simulink model "ExerciseModel_18072025"  (R2025a)
settings: Solver=ode4  StartTime=0.0  StopTime=tsim  FixedStep=1  RelTol=1e-3
model workspace (MAT data in the model file):
  step_size = 1
values from neighbouring files (symbols this model uses):
  A_w = [cosd(beta1)*sind(alfa1)  -cosd(beta2)*sind(alfa2) -cosd(beta3)*sind(alfa3) cosd(beta4)*sind(alfa4) ... (first row only)    [initfun_18072025.m]    (also in initfun_18072025_nogyro.m)
  A_wP = pinv(A_w)    [initfun_18072025.m]    (also in initfun_18072025_nogyro.m)
  ARW = deg2rad(0.23)/sqrt(3600)    [initfun_18072025.m]
  Bias = deg2rad(1)/3600    [initfun_18072025.m]
  C_d = 2.2    [initfun_18072025.m]    (also in initfun_18072025_nogyro.m)
  d_max = 0.29    [initfun_18072025.m]    (also in initfun_18072025_nogyro.m)
  d_min = 0    [initfun_18072025.m]    (also in initfun_18072025_nogyro.m)
  ET0 = cspice_str2et(Date_UTC)    [initfun_18072025.m]    (also in initfun_18072025_nogyro.m)
  FOV = 166    [initfun_18072025.m]    (also in initfun_18072025_nogyro.m)
  G_earth = 6.6742e-11    [initfun_18072025.m]    (also in initfun_18072025_nogyro.m)
  init_state = [initial_position,initial_velocity,ang_vel_init2,quat_0]'    [initfun_18072025.m]    (also in initfun_18072025_nogyro.m)
  K = [F Z(:); Z(:)' sigma]    [Gain_matrix.m]    (also in QUEST.m = Gain_matrix(V',W',a); initfun_18072025.m = schmidt(nmax, mmax); initfun_18072025_nogyro.m = schmidt(nmax, mmax))
  K_dp = K_d_pitch_1    [evaluate_gains.m]    (also in evaluate_gains_nogyro.m)
  K_dr = K_d_roll_1    [evaluate_gains.m]    (also in evaluate_gains_nogyro.m)
  K_dy = K_d_yaw_1    [evaluate_gains.m]    (also in evaluate_gains_nogyro.m)
  K_pp = K_p_pitch_1    [evaluate_gains.m]    (also in evaluate_gains_nogyro.m; initfun_18072025_nogyro.m = K_pp/2)
  K_pr = K_p_roll_1    [evaluate_gains.m]    (also in evaluate_gains_nogyro.m; initfun_18072025.m = K_pr*1.8)
  K_py = K_p_yaw_1    [evaluate_gains.m]    (also in evaluate_gains_nogyro.m; initfun_18072025.m = K_py*10)
  m_earth = 5.9736e24    (= 5.9736e+24)    [initfun_18072025.m]    (also in initfun_18072025_nogyro.m)
  Magnetic_dipole = [0.1; 0.1;  0.1]    [initfun_18072025.m]    (also in initfun_18072025_nogyro.m)
  Magnetometers_number = 2    [initfun_18072025.m]    (also in initfun_18072025_nogyro.m)
  Mean_cart_Mag = 0    [initfun_18072025.m]    (also in initfun_18072025_nogyro.m)
  MeanangularSun = 0    [initfun_18072025.m]    (also in initfun_18072025_nogyro.m)
  mmax = 3    [initfun_18072025.m]    (also in initfun_18072025_nogyro.m)
  nmax = 3    [initfun_18072025.m]    (also in initfun_18072025_nogyro.m)
  omegaOrb = [0;-2*pi/P;0]    [initfun_18072025.m]    (also in initfun_18072025_nogyro.m)
  P_prev = [P_dg, zeros(3,3) ... (first row only)    [initfun_18072025.m]    (also in initfun_18072025_nogyro.m)
  P_sun = 4.56e-6    (= 4.56e-06)    [initfun_18072025.m]    (also in initfun_18072025_nogyro.m)
  Q = [eye(3,3).*Qattitudefactor zeros(3,3) ... (first row only)    [initfun_18072025.m]    (also in initfun_18072025_nogyro.m)
  R_B = (Sigma_cart_Mag)^2    (= 2.77777777778e-16)    [initfun_18072025.m]    (also in initfun_18072025_nogyro.m)
  r_earth = 6371e3    (= 6371000)    [initfun_18072025.m]    (also in initfun_18072025_nogyro.m)
  R_G = ARW^2    [initfun_18072025.m]
  R_SS = (SigmaangularSun*pi/180)^2    (= 3.04617419787e-06)    [initfun_18072025.m]    (also in initfun_18072025_nogyro.m)
  RWs_Inertia = diag([9.0718e-06, 9.0718e-06, 9.0718e-06, 9.0718e-06])    [initfun_18072025.m]    (also in initfun_18072025_nogyro.m)
  RWs_Inertia_Inv = inv(RWs_Inertia)    [initfun_18072025.m]    (also in initfun_18072025_nogyro.m)
  Sat_Inertia = diag([6.295, 1.644, 5.462]*10^-1)    [initfun_18072025.m]    (also in initfun_18072025_nogyro.m)
  Sat_mass = 12.172    [initfun_18072025.m]    (also in initfun_18072025_nogyro.m)
  Sigma_cart_Mag = (50*10^-9)/3    (= 1.66666666667e-08)    [initfun_18072025.m]    (also in initfun_18072025_nogyro.m)
  SigmaangularSun = 0.1    [initfun_18072025.m]    (also in initfun_18072025_nogyro.m)
  Sun_sensors = zeros(3, SS_number)    [initfun_18072025.m]    (also in initfun_18072025_nogyro.m)
  threshold_omega = omega_max * 0.8    (= 837.7580408)    [initfun_18072025.m]    (also in initfun_18072025_nogyro.m)
  x_prev = x0    [initfun_18072025.m]    (also in initfun_18072025_nogyro.m)
undefined symbols (not defined in the file or in its folder): DiscIntNeverNeededParam, G, H, IAU, juliandate, quat_feed_reg, Sat_Aeromodel_det
libraries: matrix_library x9, vrlib x2, aerolibtransform2 x1
(part 2 of 3)

== system ExerciseModel_18072025/External Disturbance Torques/Magnetic Torque ==
  POS_ECI [km] : Inport
  R(IRF->BRF) : Inport  Port=2
  Cross Product : matrix_library/Cross Product
  Earth magnetc Field : Subsystem
  m : Constant  Value=Magnetic_dipole
  T_mag : Outport
  B : Outport  Port=2
  IRF Earth magnetic field (T) : Outport  Port=3
  wires:
  POS_ECI [km]/1 -> Earth magnetc Field/1(R_ECI)
  Earth magnetc Field/1("BRF Earth magnetic field (T)  ") -> Cross Product/2, B/1
  m/1 -> Cross Product/1
  Cross Product/1 -> T_mag/1
  R(IRF->BRF)/1 -> Earth magnetc Field/2(R(IRF->BRF))
  Earth magnetc Field/2(IRF Earth magnetic field (T)) -> IRF Earth magnetic field (T)/1

== system ExerciseModel_18072025/External Disturbance Torques/SRP_torque_evaluation ==
  Sdir_eci_vec : Inport
  R_ECIBRF : Inport  Port=2
  eclipse_flag : Inport  Port=3
  Constant : Constant  Value=P_sun
  SRP1 : MATLAB Function  TreatAsAtomicUnit=on  SystemSampleTime=step_size
  To Workspace : ToWorkspace  VariableName=srp_torque  SaveFormat=Timeseries  SampleTime=-1
  To Workspace1 : ToWorkspace  VariableName=torque_contrib  SaveFormat=Timeseries  SampleTime=-1
  torque_SRP : Outport
  wires:
  Sdir_eci_vec/1 -> SRP1/1(Sdir_ECI_vec)
  R_ECIBRF/1 -> SRP1/2(R_ECIBRF)
  SRP1/1(torque) -> To Workspace/1, torque_SRP/1
  eclipse_flag/1 -> SRP1/3(eclipse_flag)
  Constant/1 -> SRP1/4(P_sun)
  SRP1/2(torque_contribution) -> To Workspace1/1

== system ExerciseModel_18072025/Performance Block /Altitude Check ==
  In1 : Inport
  Constant : Constant  Value=r_earth*10^-3
  Dot Product : DotProduct  OutDataTypeStr=Inherit: Inherit via internal rule
  Scope : Scope
      settings: ActiveDisplayYMinimum=615.9620311742791  ActiveDisplayYMaximum=646.34171943145168
  Square Root : Sqrt
  Subtract : Sum  Inputs=+-
  wires:
  In1/1 -> Dot Product/1, Dot Product/2
  Constant/1 -> Subtract/2
  Square Root/1 -> Subtract/1
  Dot Product/1 -> Square Root/1
  Subtract/1 -> Scope/1

== system ExerciseModel_18072025/Performance Block /Mo ==
  X (km) [ECI] : Inport
  V (km/s) [ECI] : Inport  Port=2
  MATLAB Function : MATLAB Function  TreatAsAtomicUnit=on
  Transpose : Math  Operator=transpose
  Out1 : Outport
  wires:
  Transpose/1 -> Out1/1
  MATLAB Function/1(Mo) -> Transpose/1
  X (km) [ECI]/1 -> MATLAB Function/1(X)
  V (km/s) [ECI]/1 -> MATLAB Function/2(V)

== system ExerciseModel_18072025/Actuators/RW simplified model/Subsystem ==
  omega_old : Inport
  Constant1 : Constant  Value=RWs_Inertia
  Constant2 : Constant  Value=A_w
  Demux2 : Demux
  Matrix Multiply1 : Product  Multiplication=Matrix(*)
  Matrix Multiply2 : Product  Multiplication=Matrix(*)
  Scope1 : Scope  NumInputPorts=4
      settings: ActiveDisplayYMinimum=-0.0627  ActiveDisplayYMaximum=0.0755
  To Workspace : ToWorkspace  VariableName=h_wheels2  SaveFormat=Structure  SampleTime=-1
      settings: Save2DSignal=2-D array (concatenate along first dimension)
  To Workspace2 : ToWorkspace  VariableName=h_wheels3  SaveFormat=Structure  SampleTime=-1
      settings: Save2DSignal=2-D array (concatenate along first dimension)
  Transpose : Math  Operator=transpose
  hw_w : Outport
  Hw_4w : Outport  Port=2
  wires:
  Transpose/1 -> To Workspace/1
  Matrix Multiply2/1 -> hw_w/1
  Constant2/1 -> Matrix Multiply2/1
  Demux2/1 -> Scope1/1
  Demux2/4 -> Scope1/4
  Constant1/1 -> Matrix Multiply1/1
  Matrix Multiply1/1 -> Matrix Multiply2/2, To Workspace2/1, Transpose/1, Hw_4w/1, Demux2/1
  Demux2/2 -> Scope1/2
  Demux2/3 -> Scope1/3
  omega_old/1 -> Matrix Multiply1/2

== system ExerciseModel_18072025/Discrete Drag in ECI/DRAG FORCE IN ORF [N]/AREA LOOK-UP ==
  roll : Inport
  pitch angle : Inport  Port=2
  yaw angle : Inport  Port=3
  MATLAB Function : MATLAB Function  TreatAsAtomicUnit=on
  Merge : Merge
  Scope2 : Scope
      settings: ActiveDisplayYMinimum=-0.588573963748372  ActiveDisplayYMaximum=0.52172797483263089  DataLoggingVariableName=ScopeData26
  Subsystem : Subsystem
  Subsystem1 : Subsystem
  Area : Outport
  wires:
  Merge/1 -> Area/1, Scope2/1
  Subsystem1/1(Area) -> Merge/2
  MATLAB Function/2(out2) -> Subsystem1/Enable
  MATLAB Function/1(out1) -> Subsystem/Enable
  yaw angle/1 -> Subsystem/3(yaw angle), Subsystem1/3(yaw angle), MATLAB Function/3(yaw_angle)
  pitch angle/1 -> MATLAB Function/2(pitch_angle), Subsystem/2(pitch angle), Subsystem1/2(pitch angle)
  roll/1 -> MATLAB Function/1(roll_angle), Subsystem/1(roll), Subsystem1/1(roll)
  Subsystem/1(Area) -> Merge/1

== system ExerciseModel_18072025/External Disturbance Torques/AeroTorque in BRF/TORQUE FACTOR ==
  roll : Inport
  pitch angle : Inport  Port=2
  yaw angle : Inport  Port=3
  MATLAB Function : MATLAB Function  TreatAsAtomicUnit=on
  Merge : Merge
  Subsystem : Subsystem
  Subsystem1 : Subsystem
  T_comp : Outport
  wires:
  Subsystem1/1(T_components) -> Merge/2
  Merge/1 -> T_comp/1
  Subsystem/1(T_components) -> Merge/1
  MATLAB Function/2(out2) -> Subsystem1/Enable
  MATLAB Function/1(out1) -> Subsystem/Enable
  yaw angle/1 -> MATLAB Function/3(yaw_angle), Subsystem/3(yaw angle), Subsystem1/3(yaw angle)
  pitch angle/1 -> MATLAB Function/2(pitch_angle), Subsystem/2(pitch angle), Subsystem1/2(pitch angle)
  roll/1 -> MATLAB Function/1(roll_angle), Subsystem/1(roll), Subsystem1/1(roll)

== system ExerciseModel_18072025/External Disturbance Torques/Magnetic Torque/Earth magnetc Field ==
  R_ECI : Inport
  R(IRF->BRF) : Inport  Port=2
  Clock : Clock
  Direction Cosine Matrix ECI to ECEF : aerolibtransform2/Direction Cosine Matrix ECI to ECEF  red=IAU-2000/2006  year=2025  month=July  day=23  hour=8  min=30  sec=0  deltaT=Sec  errorflag=Error  extraparamflag=off
      settings: AttributesFormatString=%<red>
  "Earth magnetic field " : MATLAB Function  TreatAsAtomicUnit=on
  G : Constant  Value=G  VectorParams1D=off
  H : Constant  Value=H  VectorParams1D=off
  K : Constant  Value=K  VectorParams1D=off
  Math Function : Math  Operator=transpose  SignedPower=on
  Matrix Multiply : Product  Multiplication=Matrix(*)
  Matrix Multiply1 : Product  Multiplication=Matrix(*)
  Matrix Multiply2 : Product  Multiplication=Matrix(*)
  "Maximum degree of harmonics " : Constant  Value=mmax
  "Maximum order of harmonics " : Constant  Value=nmax
  Reshape : Reshape  OutputDimensionality=Column vector (2-D)
  Reshape1 : Reshape  OutputDimensionality=Column vector (2-D)
  Scope : Scope
      settings: ActiveDisplayYMinimum=-5.8566873314651838E-5  ActiveDisplayYMaximum=5.7983261253001576E-5  DataLoggingVariableName=ScopeData41
  "BRF Earth magnetic field (T)  " : Outport
  IRF Earth magnetic field (T) : Outport  Port=2
  wires:
  R(IRF->BRF)/1 -> Matrix Multiply/1
  Matrix Multiply/1 -> "BRF Earth magnetic field (T)  "/1, Scope/1
  Math Function/1 -> Matrix Multiply1/1
  "Earth magnetic field "/1(B) -> Reshape1/1
  Matrix Multiply2/1 -> "Earth magnetic field "/1(r_ECEF)
  Direction Cosine Matrix ECI to ECEF/1 -> Matrix Multiply2/1, Math Function/1
  Matrix Multiply1/1 -> Matrix Multiply/2, IRF Earth magnetic field (T)/1
  Clock/1 -> Direction Cosine Matrix ECI to ECEF/1
  H/1 -> "Earth magnetic field "/6(H)
  "Maximum order of harmonics "/1 -> "Earth magnetic field "/2(nmax)
  "Maximum degree of harmonics "/1 -> "Earth magnetic field "/3(mmax)
  G/1 -> "Earth magnetic field "/5(G)
  K/1 -> "Earth magnetic field "/4(K)
  Reshape/1 -> Matrix Multiply2/2
  Reshape1/1 -> Matrix Multiply1/2
  R_ECI/1 -> Reshape/1

== system ExerciseModel_18072025/Discrete Drag in ECI/DRAG FORCE IN ORF [N]/AREA LOOK-UP/Subsystem ==
  roll : Inport
  pitch angle : Inport  Port=2
  yaw angle : Inport  Port=3
  Enable : EnablePort
  Scope : Scope
      settings: ActiveDisplayYMinimum=-17087.602647570646  ActiveDisplayYMaximum=29156.954716718436  DataLoggingVariableName=ScopeData24
  n-D Lookup Table2 : Lookup_n-D  NumberOfTableDimensions=3  BreakpointsForDimension1=Sat_Aeromodel_det.roll  BreakpointsForDimension2=Sat_Aeromodel_det.pitch  BreakpointsForDimension3=Sat_Aeromodel_det.yaw  Table=Sat_Aeromodel_det.Area  InterpMethod=Cubic spline  ExtrapMethod=Cubic spline  InternalRulePriority=Speed  RndMeth=Simplest
      settings: InputPortMap=u0,u1,u2
  Area : Outport
  wires:
  pitch angle/1 -> n-D Lookup Table2/2
  roll/1 -> n-D Lookup Table2/1
  yaw angle/1 -> n-D Lookup Table2/3
  n-D Lookup Table2/1 -> Scope/1, Area/1

== system ExerciseModel_18072025/Discrete Drag in ECI/DRAG FORCE IN ORF [N]/AREA LOOK-UP/Subsystem1 ==
  roll : Inport
  pitch angle : Inport  Port=2
  yaw angle : Inport  Port=3
  Enable : EnablePort
  Scope1 : Scope
      settings: ActiveDisplayYMinimum=-0.41348067878016787  ActiveDisplayYMaximum=0.34441355379815991  DataLoggingVariableName=ScopeData25
  n-D Lookup Table2 : Lookup_n-D  NumberOfTableDimensions=3  BreakpointsForDimension1=Sat_Aeromodel_det.roll  BreakpointsForDimension2=Sat_Aeromodel_det.pitch  BreakpointsForDimension3=Sat_Aeromodel_det.yaw  Table=Sat_Aeromodel_det.Area  InterpMethod=Cubic spline  ExtrapMethod=Cubic spline  InternalRulePriority=Speed  RndMeth=Simplest
      settings: InputPortMap=u0,u1,u2
  Area : Outport
  wires:
  pitch angle/1 -> n-D Lookup Table2/2
  roll/1 -> n-D Lookup Table2/1
  yaw angle/1 -> n-D Lookup Table2/3
  n-D Lookup Table2/1 -> Scope1/1, Area/1

== system ExerciseModel_18072025/External Disturbance Torques/AeroTorque in BRF/TORQUE FACTOR/Subsystem ==
  roll : Inport
  pitch angle : Inport  Port=2
  yaw angle : Inport  Port=3
  Enable : EnablePort
  Mux : Mux  Inputs=3
  Scope : Scope
      settings: ActiveDisplayYMinimum=-8.30252  ActiveDisplayYMaximum=7.64736
  n-D Lookup Table : Lookup_n-D  NumberOfTableDimensions=3  BreakpointsForDimension1=Sat_Aeromodel_det.roll  BreakpointsForDimension2=Sat_Aeromodel_det.pitch  BreakpointsForDimension3=Sat_Aeromodel_det.yaw  Table=Sat_Aeromodel_det.xComp  InterpMethod=Cubic spline  ExtrapMethod=Cubic spline  InternalRulePriority=Speed  RndMeth=Simplest
      settings: InputPortMap=u0,u1,u2
  n-D Lookup Table1 : Lookup_n-D  NumberOfTableDimensions=3  BreakpointsForDimension1=Sat_Aeromodel_det.roll  BreakpointsForDimension2=Sat_Aeromodel_det.pitch  BreakpointsForDimension3=Sat_Aeromodel_det.yaw  Table=Sat_Aeromodel_det.yComp  InterpMethod=Cubic spline  ExtrapMethod=Cubic spline  InternalRulePriority=Speed  RndMeth=Simplest
      settings: InputPortMap=u0,u1,u2
  n-D Lookup Table2 : Lookup_n-D  NumberOfTableDimensions=3  BreakpointsForDimension1=Sat_Aeromodel_det.roll  BreakpointsForDimension2=Sat_Aeromodel_det.pitch  BreakpointsForDimension3=Sat_Aeromodel_det.yaw  Table=Sat_Aeromodel_det.zComp  InterpMethod=Cubic spline  ExtrapMethod=Cubic spline  InternalRulePriority=Speed  RndMeth=Simplest
      settings: InputPortMap=u0,u1,u2
  T_components : Outport
  wires:
  yaw angle/1 -> n-D Lookup Table/3, n-D Lookup Table1/3, n-D Lookup Table2/3
  pitch angle/1 -> n-D Lookup Table/2, n-D Lookup Table1/2, n-D Lookup Table2/2
  roll/1 -> n-D Lookup Table/1, n-D Lookup Table1/1, n-D Lookup Table2/1
  n-D Lookup Table2/1 -> Mux/3
  Mux/1 -> T_components/1, Scope/1
  n-D Lookup Table/1 -> Mux/1
  n-D Lookup Table1/1 -> Mux/2

== system ExerciseModel_18072025/External Disturbance Torques/AeroTorque in BRF/TORQUE FACTOR/Subsystem1 ==
  roll : Inport
  pitch angle : Inport  Port=2
  yaw angle : Inport  Port=3
  Enable : EnablePort
  Mux : Mux  Inputs=3
  Scope : Scope
      settings: ActiveDisplayYMinimum=-0.00141  ActiveDisplayYMaximum=0.00246  DataLoggingVariableName=ScopeData2
  n-D Lookup Table : Lookup_n-D  NumberOfTableDimensions=3  BreakpointsForDimension1=Sat_Aeromodel_det.roll  BreakpointsForDimension2=Sat_Aeromodel_det.pitch  BreakpointsForDimension3=Sat_Aeromodel_det.yaw  Table=Sat_Aeromodel_det.xComp  InterpMethod=Cubic spline  ExtrapMethod=Cubic spline  InternalRulePriority=Speed  RndMeth=Simplest
      settings: InputPortMap=u0,u1,u2
  n-D Lookup Table1 : Lookup_n-D  NumberOfTableDimensions=3  BreakpointsForDimension1=Sat_Aeromodel_det.roll  BreakpointsForDimension2=Sat_Aeromodel_det.pitch  BreakpointsForDimension3=Sat_Aeromodel_det.yaw  Table=Sat_Aeromodel_det.yComp  InterpMethod=Cubic spline  ExtrapMethod=Cubic spline  InternalRulePriority=Speed  RndMeth=Simplest
      settings: InputPortMap=u0,u1,u2
  n-D Lookup Table2 : Lookup_n-D  NumberOfTableDimensions=3  BreakpointsForDimension1=Sat_Aeromodel_det.roll  BreakpointsForDimension2=Sat_Aeromodel_det.pitch  BreakpointsForDimension3=Sat_Aeromodel_det.yaw  Table=Sat_Aeromodel_det.zComp  InterpMethod=Cubic spline  ExtrapMethod=Cubic spline  InternalRulePriority=Speed  RndMeth=Simplest
      settings: InputPortMap=u0,u1,u2
  T_components : Outport
  wires:
  yaw angle/1 -> n-D Lookup Table/3, n-D Lookup Table1/3, n-D Lookup Table2/3
  pitch angle/1 -> n-D Lookup Table/2, n-D Lookup Table1/2, n-D Lookup Table2/2
  roll/1 -> n-D Lookup Table/1, n-D Lookup Table1/1, n-D Lookup Table2/1
  n-D Lookup Table2/1 -> Mux/3
  Mux/1 -> T_components/1, Scope/1
  n-D Lookup Table/1 -> Mux/1
  n-D Lookup Table1/1 -> Mux/2

== matlab function ExerciseModel_18072025/QFR/MATLAB Function ==
  data: q_c input; dq output; q input
function dq  = qmultiply(q_c,q)
%#codegen
%% Quaternion multiplication
% qs = ps*rs - pv'*rv
% qv = ps*rv + rs*pv - pv x rv
%r(1:3) = -r(1:3);
%% INPUT 
% p: vector 4x1
% r: vector 4x1

%% OUTPUT
% q: vector 4x1

% N.B. The first component of the quaternion is the scalar part
q(1:3) = -q(1:3);
% q(4) = p(4)*r(4) - p(1:3)'*r(1:3);
% q(1:3) = p(4)*r(1:3) + r(4)*p(1:3) - cross(p(1:3),r(1:3));
dqs=zeros(4,1);
dqs(1:3,1) = q_c(4)*q(1:3)+q(4)*q_c(1:3)-cross(q_c(1:3),q(1:3));
dqs(4,1) = q_c(4)*q(4)-q_c(1:3)'*q(1:3);
dq = sign(dqs(4))*dqs(1:3);
appo = q(1:4);
end

== matlab function ExerciseModel_18072025/QFR/ECI  to ORF ==
  data: q input; R output
function R = R_by_q(q)

%% Description 
% This block provides the rotation matrix corresponding to the quaternion
% in input. THE SCALAR LAST CONVENTION IS USED FOR THE QUATERNION

%% INPUT 
% q -> 4x1 array (quaternion)
%% OUTPUT 
% R -> 3x3 matrix (rotation matrix)
q0 = q(4); 
q1 = q(1);
q2 = q(2);
q3 = q(3);

R = [q0^2+q1^2-q2^2-q3^2 2*q1*q2+2*q0*q3 2*q1*q3-2*q0*q2;
    2*q1*q2-2*q0*q3 q0^2-q1^2+q2^2-q3^2 2*q2*q3+2*q0*q1;
    2*q1*q3+2*q0*q2 2*q2*q3-2*q0*q1 q0^2-q1^2-q2^2+q3^2];
end

== matlab function ExerciseModel_18072025/External Disturbance Torques/AeroTorque in BRF/TORQUE FACTOR/MATLAB Function ==
  data: roll_angle input; out1 output; pitch_angle input; yaw_angle input; out2 output
function [out1, out2]= aero_selection(roll_angle, pitch_angle, yaw_angle)


if abs(roll_angle)>0.2618
    out1=1;
    out2=0;

else if abs(pitch_angle)>0.2618

        out1=1;
        out2=0;
else if abs(yaw_angle)>0.2618

        out1=1;
        out2=0;
else
    out1=0;
    out2=1;
end
end
end
end

== matlab function ExerciseModel_18072025/QFR/ECI to BRF ==
  data: q input; R output
function R = R_by_q(q)

%% Description 
% This block provides the rotation matrix corresponding to the quaternion
% in input. THE SCALAR LAST CONVENTION IS USED FOR THE QUATERNION

%% INPUT 
% q -> 4x1 array (quaternion)
%% OUTPUT 
% R -> 3x3 matrix (rotation matrix)
q0 = q(4); 
q1 = q(1);
q2 = q(2);
q3 = q(3);

R = [q0^2+q1^2-q2^2-q3^2 2*q1*q2+2*q0*q3 2*q1*q3-2*q0*q2;
    2*q1*q2-2*q0*q3 q0^2-q1^2+q2^2-q3^2 2*q2*q3+2*q0*q1;
    2*q1*q3+2*q0*q2 2*q2*q3-2*q0*q1 q0^2-q1^2-q2^2+q3^2];
end

== matlab function ExerciseModel_18072025/Discrete Drag in ECI/DRAG FORCE IN ORF [N]/AREA LOOK-UP/MATLAB Function ==
  data: roll_angle input; out1 output; pitch_angle input; yaw_angle input; out2 output
function [out1, out2]= aero_selection(roll_angle, pitch_angle, yaw_angle)


if abs(roll_angle)>0.2618
    out1=1;
    out2=0;

else if abs(pitch_angle)>0.2618

        out1=1;
        out2=0;
else if abs(yaw_angle)>0.2618

        out1=1;
        out2=0;
else
    out1=0;
    out2=1;
end
end
end
end

== matlab function ExerciseModel_18072025/MATLAB Function ==
  data: q input; R output
function R = R_by_q(q)

%% Description 
% This block provides the rotation matrix corresponding to the quaternion
% in input. THE SCALAR LAST CONVENTION IS USED FOR THE QUATERNION

%% INPUT 
% q -> 4x1 array (quaternion)
%% OUTPUT 
% R -> 3x3 matrix (rotation matrix)
q = q / norm(q); 
q0 = q(4); 
q1 = q(1);
q2 = q(2);
q3 = q(3);

R = [q0^2+q1^2-q2^2-q3^2 2*q1*q2+2*q0*q3 2*q1*q3-2*q0*q2;
    2*q1*q2-2*q0*q3 q0^2-q1^2+q2^2-q3^2 2*q2*q3+2*q0*q1;
    2*q1*q3+2*q0*q2 2*q2*q3-2*q0*q1 q0^2-q1^2-q2^2+q3^2];
end

== matlab function ExerciseModel_18072025/Quat From Rot ==
  data: dcm input; q output
function q = q_by_R(dcm)
%% Description 
% This block provides the quaternion corresponding to the rotation matrix 
% in input. THE SCALAR LAST CONVENTION IS USED FOR THE QUATERNION. 
%% INPUT 
% R -> 3x3 matrix (rotation matrix)
%% OUTPUT 
% q -> 4x1 array (quaternion)
q = zeros(4,1);
tr = trace(dcm);
 if (tr > 0)
        sqtrp1 = sqrt( tr + 1.0 );
        q(4) = 0.5*sqtrp1; 
        q(1) = (dcm(2, 3) - dcm(3, 2))/(2.0*sqtrp1);
        q(2) = (dcm(3, 1) - dcm(1, 3))/(2.0*sqtrp1); 
        q(3) = (dcm(1, 2) - dcm(2, 1))/(2.0*sqtrp1); 
    else
        d = diag(dcm(:,:));
        if ((d(2) > d(1)) && (d(2) > d(3)))
            % max value at dcm(2,2,i)
            sqdip1 = sqrt(d(2) - d(1) - d(3) + 1.0 );
            
            q(2) = 0.5*sqdip1; 
            
            if ( sqdip1 ~= 0 )
                sqdip1 = 0.5/sqdip1;
            end
            
            q(4) = (dcm(3, 1) - dcm(1, 3))*sqdip1; 
            q(1) = (dcm(1, 2) + dcm(2, 1))*sqdip1; 
            q(3) = (dcm(2, 3) + dcm(3, 2))*sqdip1; 
        elseif (d(3) > d(1))
            % max value at dcm(3,3,i)
            sqdip1 = sqrt(d(3) - d(1) - d(2) + 1.0 );
            
            q(3) = 0.5*sqdip1; 
            
            if ( sqdip1 ~= 0 )
                sqdip1 = 0.5/sqdip1;
            end
            
            q(4) = (dcm(1, 2) - dcm(2, 1))*sqdip1;
            q(1) = (dcm(3, 1) + dcm(1, 3))*sqdip1; 
            q(2) = (dcm(2, 3) + dcm(3, 2))*sqdip1; 
        else
            % max value at dcm(1,1,i)
            sqdip1 = sqrt(d(1) - d(2) - d(3) + 1.0 );
            
            q(1) = 0.5*sqdip1; 
            
            if ( sqdip1 ~= 0 )
                sqdip1 = 0.5/sqdip1;
            end
            
            q(4) = (dcm(2, 3) - dcm(3, 2))*sqdip1; 
            q(2) = (dcm(1, 2) + dcm(2, 1))*sqdip1; 
            q(3) = (dcm(3, 1) + dcm(1, 3))*sqdip1; 
        end
 end 

end

== matlab function ExerciseModel_18072025/Sensors/Angular velocity noise ==
  data: omega_true input; Bias_omega input; ARW input; dt input; omega_noise output
function omega_noise  = noiseOmega(omega_true, Bias_omega, ...
    ARW, dt)

omega_noise = zeros(3,1);
omega_noise = omega_true(:) + Bias_omega + randn(3,1)*ARW/sqrt(dt);

end

== matlab function ExerciseModel_18072025/Performance Block /R(IRF->BRF) ==
  data: q input; R output
function R = R_by_q(q)

%% Description 
% This block provides the rotation matrix corresponding to the quaternion
% in input. THE SCALAR LAST CONVENTION IS USED FOR THE QUATERNION

%% INPUT 
% q -> 4x1 array (quaternion)
%% OUTPUT 
% R -> 3x3 matrix (rotation matrix)
q = q / norm(q); 
q0 = q(4); 
q1 = q(1);
q2 = q(2);
q3 = q(3);

R = [q0^2+q1^2-q2^2-q3^2 2*q1*q2+2*q0*q3 2*q1*q3-2*q0*q2;
    2*q1*q2-2*q0*q3 q0^2-q1^2+q2^2-q3^2 2*q2*q3+2*q0*q1;
    2*q1*q3+2*q0*q2 2*q2*q3-2*q0*q1 q0^2-q1^2-q2^2+q3^2];
end

== matlab function ExerciseModel_18072025/Actuators/RW simplified model/MATLAB Function ==
  data: omega_dot input; threshold_omega input; omega output; omega_old input; omega_dot_new output
function [omega, omega_dot_new] = omega_new(omega_dot, threshold_omega, omega_old)
t=1;
omega=omega_dot*t+omega_old;

for i = 1:4
    if abs(omega(i)) > threshold_omega
        omega(i) = sign(omega(i))*threshold_omega;
    end
end

omega_dot_new = (omega - omega_old)*(1/t);

== matlab function ExerciseModel_18072025/Performance Block /Mo/MATLAB Function ==
  data: X input; Mo output; V input
function Mo = ECI_to_ORF(X,V)

A=cross(cross(-X,V),-X);
B=norm(A); % A/B is i_0 

C=cross(-X,V);
D=norm(C); % C/D is j_0

E=-X;
F=norm(X); % E/F is i_0

Mo=[A(1)/B  A(2)/B  A(3)/B;
    
    C(1)/D  C(2)/D  C(3)/D;
    
    E(1)/F  E(2)/F  E(3)/F];


end

== matlab function ExerciseModel_18072025/Discrete Drag in ECI/DRAG FORCE IN ORF [N]/MATLAB Function ==
  data: z input; density output
% ATMOSPHERE calculates density for altitudes from sea level
% through 1000 km using exponential interpolation.
%wwwwwwwwwwwwwwwwwwwwwwwwwwwwwwwwwwwwwwwwwwwwwwwww
%function density = atmosphere(z)
%z[km]
function density = atmosphere(z)
%...Geometric altitudes (km):
h = ...
[ 0 25 30 40 50 60 70 ...
80 90 100 110 120 130 140 ...
150 180 200 250 300 350 400 ...
450 500 600 700 800 900 1000];
%...Corresponding densities (kg/m^3) from USSA76:
r = ...
[1.225 4.008e-2 1.841e-2 3.996e-3 1.027e-3 3.097e-4 8.283e-5 ...
1.846e-5 3.416e-6 5.606e-7 9.708e-8 2.222e-8 8.152e-9 3.831e-9 ...
2.076e-9 5.194e-10 2.541e-10 6.073e-11 1.916e-11 7.014e-12 2.803e-12 ...
1.184e-12 5.215e-13 1.137e-13 3.070e-14 1.136e-14 5.759e-15 3.561e-15];
%...Scale heights (km):
H = ...
[ 7.310 6.427 6.546 7.360 8.342 7.583 6.661 ...
5.927 5.533 5.703 6.782 9.973 13.243 16.322 ...
21.652 27.974 34.934 43.342 49.755 54.513 58.019 ...
60.980 65.654 76.377 100.587 147.203 208.020];
%...Handle altitudes outside of the range:

if z > 1000
z = 1000;
elseif z < 0
z = 0;
end

i=0;  %initialize i

%...Determine the interpolation interval:
for j = 1:27
if z >= h(j) && z < h(j+1)
i = j;
end
end
if z == 1000
i = 27;
end
%...Exponential interpolation:
density = r(i)*exp(-(z - h(i))/H(i));
end %atmosphere
% %wwwwwwwwwwwwwwwwwwwwwwwwwwwwwwwwwwwwwwwwwwwwwwwww
%

== matlab function ExerciseModel_18072025/Sensors/Sun direction noise ==
  data: Sdir_BRF_matrix input; Sdir_BRF_matrix_noise output; MeanangularSun input; SigmaangularSun input
function Sdir_BRF_matrix_noise = noiseSun(Sdir_BRF_matrix, MeanangularSun, ...
    SigmaangularSun)


sizeS = size(Sdir_BRF_matrix);
s = sizeS(2);

if s == 0
    Sdir_BRF_matrix_noise = [];
else
    Sdir_BRF_matrix_noise = zeros(sizeS);
    
    s_true = Sdir_BRF_matrix(:,1);
    s_true = s_true(:);
    
    for i = 1:s   
        Alpha_s=deg2rad(MeanangularSun)+randn(1).*deg2rad(SigmaangularSun); %radians
        Beta_s=rand(1).*2*pi; %radians
    
        if s_true==[1;0;0]    
            k_s=[0 0 1]';
        else
            k_s=[1 0 0]';
        end
        
        h_s=cross(s_true,k_s)./norm(cross(s_true,k_s));
        g_s=s_true.*cos(Alpha_s)+cross(h_s,s_true).*sin(Alpha_s);
        s_mes=g_s.*cos(Beta_s)+cross(s_true,g_s).*sin(Beta_s)+s_true.*dot(s_true,g_s).*(1-cos(Beta_s));
    
        if norm(s_mes)-1 >10e-10    
            disp('warning')
            s_mes = s_mes/norm(s_mes);
        end
    
        Sdir_BRF_matrix_noise(:,i) = s_mes/norm(s_mes); 
    end
end

== matlab function ExerciseModel_18072025/Sensors/Magnetic field noise ==
  data: B_BRF_matrix input; Mean_cart_Mag input; Sigma_cart_Mag input; B_BRF_matrix_noise output; Bdir_BRF_matrix_noise output
function [B_BRF_matrix_noise, Bdir_BRF_matrix_noise] = noiseMag(B_BRF_matrix, Mean_cart_Mag, ...
    Sigma_cart_Mag)

sizeB = size(B_BRF_matrix);
t = sizeB(2);
Bdir_BRF_matrix_noise = zeros(sizeB);
B_BRF_matrix_noise = zeros (sizeB);

B_true = B_BRF_matrix(:,1);
B_true = B_true(:);
B_meas = zeros(3,1);

for j = 1:t 
    B_meas = B_BRF_matrix(:,j) + randn(3,1)*Sigma_cart_Mag;
    B_BRF_matrix_noise(:,j) = B_meas;
    Bdir_BRF_matrix_noise(:,j) = B_meas / norm(B_meas);
end
end

== matlab function ExerciseModel_18072025/S direction, B components in BRF and ECI/MATLAB Function ==
  data: Sdir_ECI_vec input; R_ECIBRF input; Sdir_ECI_matrix output; Sdir_BRF_matrix output; Sun_sensors input; FOV input; eclipse_flag input
function [Sdir_ECI_matrix, Sdir_BRF_matrix] = fcn(Sdir_ECI_vec, R_ECIBRF, ...
    Sun_sensors, FOV, eclipse_flag)

if eclipse_flag == 0
    Sdir_ECI_matrix = [];
    Sdir_BRF_matrix = [];
else    
    Sdir_BRF_vec = R_ECIBRF*Sdir_ECI_vec; % Sun direction wrt satellite in the BRF
    
    temp_ECI = zeros(3,length(Sun_sensors(1,:)));
    temp_BRF = zeros(3,length(Sun_sensors(1,:)));
    visible = false(1, length(Sun_sensors(1,:))); 
    
    % Visibility check in sunlight
    for i = 1 : length(Sun_sensors(1,:))
    
        cos_theta = dot(Sdir_BRF_vec, Sun_sensors(:,i)); % where theta is the angle between the normal to the i-th Sun sensor and the Sun direction, both in the BRF
        
        if cos_theta > cosd(FOV/2)
                
                temp_BRF(:,i) = Sdir_BRF_vec/norm(Sdir_BRF_vec);
                temp_ECI(:,i) = Sdir_ECI_vec/norm(Sdir_ECI_vec);
                visible(i) = true;
        end
    end
    
    Sdir_ECI_matrix = temp_ECI(:, visible);
    Sdir_BRF_matrix = temp_BRF(:, visible);
end

end

== matlab function ExerciseModel_18072025/S direction, B components in BRF and ECI/MATLAB Function1 ==
  data: R_ECIBRF input; Bdir_ECI_matrix output; B_ECI_vec input; B_BRF_matrix output; Magnetometers_number input
function [Bdir_ECI_matrix, B_BRF_matrix] = fcn(R_ECIBRF, B_ECI_vec,...
    Magnetometers_number)

B_BRF_vec = R_ECIBRF * B_ECI_vec;

Bdir_ECI_matrix = zeros(3, Magnetometers_number);
B_BRF_matrix = zeros(3, Magnetometers_number);

for k = 1:Magnetometers_number
    Bdir_ECI_matrix(:,k) = B_ECI_vec/norm(B_ECI_vec);
    B_BRF_matrix(:,k) = B_BRF_vec;
end

end

== matlab function ExerciseModel_18072025/MEKF Performances/phierr function ==
  data: q_est input; phierr output; q_BECI input
function phierr  = fcn(q_est, q_BECI)

    dq=q_product(q_est',[-q_BECI(1:3)'; q_BECI(4)]);
    dq = dq / norm(dq);
    
    if dq(4)<0
        dq=-dq;
    end
    % if abs(1-dq(4)) < 1e-4
    %     dq(4) = 1;
    % end

    phierr = 2*acosd(dq(4));

== matlab function ExerciseModel_18072025/Actuators/RWs Power Profile Check1/MATLAB Function ==
  data: h_wh input; T_RWs output; Tw_4Comp input; T_lim output; T_lim_inf output
function [T_RWs,T_lim,T_lim_inf] = T_wheels(h_wh, Tw_4Comp)

% h_wh = RWs angular momentum (given by the integration of T_RWs);
% Tw_4Comp = RWs Torques without friction;

% RWs angular velocities;

omega=zeros(4,1);
omega(1)=h_wh(1)/0.000250;
omega(2)=h_wh(2)/0.000250;
omega(3)=h_wh(3)/0.000250;
omega(4)=h_wh(4)/0.000250;




T_RWs=zeros(4,1);
T_RWs(1)=Tw_4Comp(1);
T_RWs(2)=Tw_4Comp(2);
T_RWs(3)=Tw_4Comp(3);
T_RWs(4)=Tw_4Comp(4);


%% Final Comparison


   if h_wh(1) > 0
      T_max1 = 0.006-0.06*h_wh(1);
      T_min1 = -0.006;
   else
      T_max1 = 0.006;
      T_min1 = -0.006-0.06*h_wh(1);
   end

    if h_wh(2) > 0
      T_max2 = 0.006-0.06*h_wh(2);
      T_min2 = -0.006;
   else
      T_max2 = 0.006;
      T_min2 = -0.006-0.06*h_wh(2);
    end

   if h_wh(3) > 0
      T_max3 = 0.006-0.06*h_wh(3);
      T_min3 = -0.006;
   else
      T_max3 = 0.006;
      T_min3 = -0.006-0.06*h_wh(3);
   end

   if h_wh(4) > 0
      T_max4 = 0.006-0.06*h_wh(4);
      T_min4 = -0.006;
   else
      T_max4 = 0.006;
      T_min4 = -0.006-0.06*h_wh(4);
   end

   if T_RWs(1) > T_max1 
      T_RWs(1) = T_max1;
   end
   
   if T_RWs(1) < T_min1
      T_RWs(1) = T_min1;
   end

   if T_RWs(2) > T_max2 
      T_RWs(2) = T_max2;
   end
   
   if T_RWs(2) < T_min2
      T_RWs(2) = T_min2;
   end

   if T_RWs(3) > T_max3 
      T_RWs(3) = T_max3;
   end
   
   if T_RWs(3) < T_min3
      T_RWs(3) = T_min3;
   end

   if T_RWs(4) > T_max4 
      T_RWs(4) = T_max4;
   end
   
   if T_RWs(4) < T_min4
      T_RWs(4) = T_min4;
   end
   


    

%% Final Construction
T_RWs=[T_RWs(1);T_RWs(2);T_RWs(3);T_RWs(4)];
T_lim=[T_max1;T_max2;T_max3;T_max4];
T_lim_inf=[T_min1;T_min2;T_min3;T_min4];



end

== matlab function ExerciseModel_18072025/MEKF Performances/MATLAB Function1 ==
  data: DCM input; roll_est output; pitch_est output; yaw_est output
function [roll_est, pitch_est, yaw_est] = calc_angles(DCM)
%321 DCM ORF->BRF;

%Angles' computation from the rotation matrix 321;
pitch_est=asin(-DCM(1,3));          %pitch angle (beta);
roll_est=atan2(DCM(2,3),DCM(3,3)); %roll angle (alpha);
yaw_est=atan2(DCM(1,2),DCM(1,1));  %yaw angle (gamma);

end

== matlab function ExerciseModel_18072025/MEKF/MEKFfun ==
  data: Bdir_BRF input; q_est output; Sdir_BRF input; Bdir_ECI input; Sdir_ECI input; B_BRF_matrix_noise input; omega_meas input; omegaIB_est output; dt input; Sat_Inertia input; R_SS input; R_B input; R_G input; x_0 input; P_0 input; Q input; P_curr_plus output
function [q_est, omegaIB_est, P_curr_plus] = fcn(Bdir_BRF, Sdir_BRF, Bdir_ECI, Sdir_ECI, B_BRF_matrix_noise, omega_meas, ...
    dt, Sat_Inertia, R_SS, R_B, R_G, x_0, P_0, Q)
    
    persistent x_prev
    persistent P_prev

    if isempty(x_prev)
        x_prev = x_0;
        P_prev = P_0;
    end
    
    
    % Bdir_BRF e Sdir_BRF sono matrici 3xt e 3xs dove t ed s sono il numero 
    % di misure che si hanno a disposizione per la direzione del campo
    % magnetico e la direzione del sole (rispettivamente).
    x_curr_prior = zeros(1,7); %x_k-
    x_curr_plus = zeros(1,7); %x_k+
    J = Sat_Inertia;
    sizeB = size(Bdir_BRF);
    t = sizeB(2);
    sizeS = size(Sdir_BRF);
    s = sizeS(2);
    disp(s);
    H = zeros(3*(s+t+1),6); % se s,t sono nulli allora otteniamo una matrice vuota
    R = zeros(3*(s+t+1), 3*(s+t+1));

   
    %% PREDICTION
    % Quaternion propagation using non-linear process model (quaternion
    % kinematic relation, qdot=(1/2)omegaxq
    x_curr_prior(1:4) = propagate_quaternion_rk4(x_prev(1:4), x_prev(5:7), dt);

    % Angular velocity propagation using non-linear process model (Euler's
    % rotational dynamics equations

    
    skew_omega = [0 -x_prev(7) x_prev(6);
                   x_prev(7) 0 -x_prev(5);
                   -x_prev(6) x_prev(5) 0];
    x_curr_prior(5:7) = propagate_omega_rk4(x_prev(5:7), J, dt);
    %omega_dot = inv(J)*(-(skew_omega*(J*x_prev(5:7))));
    %x_curr_prior(5:7)= x_prev(5:7)+omega_dot.*dt; 

    % COVARIANCE propagation
    Jomega=J*x_prev(5:7);
    skew_Jomega= [0 -Jomega(3) Jomega(2);
        Jomega(3) 0 -Jomega(1);
        -Jomega(2) Jomega(1) 0];
    JacobProcess=[-skew_omega eye(3).*0.5;
        zeros(3,3) skew_omega*J+skew_Jomega];
    phi_est=eye(6,6)+dt.*JacobProcess;
    P_curr_m = phi_est*P_prev*phi_est' + Q*dt;
    
   %% H and R evaluation
   M_q_prior = [ x_curr_prior(1)^2 - (x_curr_prior(2))^2 - (x_curr_prior(3))^2 + x_curr_prior(4)^2, 2*(x_curr_prior(1)*x_curr_prior(2) + x_curr_prior(3)*x_curr_prior(4)), 2*(x_curr_prior(1)*x_curr_prior(3) - x_curr_prior(2)*x_curr_prior(4));      
                  2*(x_curr_prior(2)*x_curr_prior(1) - x_curr_prior(3)*x_curr_prior(4)), -(x_curr_prior(1))^2 + x_curr_prior(2)^2 - (x_curr_prior(3))^2 + x_curr_prior(4)^2, 2*(x_curr_prior(2)*x_curr_prior(3) + x_curr_prior(1)*x_curr_prior(4));    
                  2*(x_curr_prior(3)*x_curr_prior(1) + x_curr_prior(2)*x_curr_prior(4)), 2*(x_curr_prior(3)*x_curr_prior(2) - x_curr_prior(1)*x_curr_prior(4)), -(x_curr_prior(1))^2 - (x_curr_prior(2))^2 + (x_curr_prior(3))^2 + (x_curr_prior(4))^2] ;
 for i = 1 : s % non dà errore se s = 0
        bi = M_q_prior*Sdir_ECI(:,i);
        skew_bi = [0 -bi(3) bi(2);
                   bi(3) 0 -bi(1);
                  -bi(2) bi(1) 0];
        H((3*(i-1)+1):3*i, 1:3) = 2*skew_bi;
        R(3*i - 2, 3*i - 2) = R_SS;
        R(3*i - 1, 3*i - 1) = R_SS;
        R(3*i, 3*i) = R_SS;
    end

    for i = s+1 : s+t 
        bi = M_q_prior*Bdir_ECI(:,i-s);
        skew_bi = [0 -bi(3) bi(2);
                   bi(3) 0 -bi(1);
                  -bi(2) bi(1) 0];
        H((3*(i-1)+1):3*i, 1:3) = 2*skew_bi;
        R(3*i - 2, 3*i - 2) = R_B / (norm(B_BRF_matrix_noise(:,i-s)))^2;
        R(3*i - 1, 3*i - 1) = R_B / (norm(B_BRF_matrix_noise(:,i-s)))^2;
        R(3*i, 3*i) = R_B / (norm(B_BRF_matrix_noise(:,i-s)))^2;
    end
    
    H(3*(s+t)+1:3*(s+t)+3,4:6) = eye(3);
    R(3*(s+t)+1:3*(s+t)+3, 3*(s+t)+1:3*(s+t)+3) = eye(3)*R_G;
    %% CORRECTION
    % Kalman gain computation
    % if mod(i, Nstep) == 0'
        K = P_curr_m*H'*(H*P_curr_m*H'+ R)^(-1); % 6x3(s+t+1) la R deve essere quella giusta, ci dobbiamo prendere le righe e le colonne giuste di R nel workspace.
                                                                                       
    % else
    %     K=zeros(6,6);
    % end

    % Innovation computation
    hk_min = zeros(3*(s+t+1),1);
    for i = 1 : s
      hk_min((3*(i-1)+1):3*i) = M_q_prior*Sdir_ECI(:,i);
    end

    for i = s+1 : s+t 
        hk_min((3*(i-1)+1):3*i) = M_q_prior*Bdir_ECI(:,i-s);
    end
    
    hk_min(3*(s+t)+1:3*(s+t)+3) = x_curr_prior(5:7);

    delta_inn = K*([Sdir_BRF(:); Bdir_BRF(:); omega_meas(:)] - hk_min); % 6x1       
    delta_g_inn = delta_inn(1:3);
    delta_omega_inn = delta_inn(4:6);
    
    % State vector correction attitude
    delta_q_up = [delta_g_inn;1]*(1/sqrt(1+delta_g_inn'*delta_g_inn));
    x_curr_plus(1:4) = q_product(delta_q_up, x_curr_prior(1:4)');
    x_curr_plus(1:4) = x_curr_plus(1:4)/norm(x_curr_plus(1:4));
    % angular velocity
    x_curr_plus(5:7)= delta_omega_inn + x_curr_prior(5:7)';

    % COVARIANCE update
    P_curr_plus = (eye(6,6)-K*H)*P_curr_m;
    if P_curr_plus(1,1) < 0
            P_curr_plus(1,1) = 0;
    end
    

    % reset
    x_prev=x_curr_plus';
    P_prev=P_curr_plus;

    q_est = x_curr_plus(1:4);
    omegaIB_est = x_curr_plus(5:7);

    % dq=q_product(q_est(i,:)',[-q(i,1:3)';q(i,4)]); if dq(4)<0
    %     dq=-dq; end
    % phierr(i)=2*acosd(dq(4));
    %sigma_state_vector(i,:)=[sqrt(P_curr_plus(1,1))
    %sqrt(P_curr_plus(2,2)) sqrt(P_curr_plus(3,3))
    %sqrt(P_curr_plus(4,4)) sqrt(P_curr_plus(5,5))
    %sqrt(P_curr_plus(6,6))];

    end

== matlab function ExerciseModel_18072025/External Disturbance Torques/SRP_torque_evaluation/SRP1 ==
  data: Sdir_ECI_vec input; R_ECIBRF input; torque output; eclipse_flag input; P_sun input; torque_contribution output
function [torque, torque_contribution] = fcn(Sdir_ECI_vec, R_ECIBRF, eclipse_flag, P_sun)
% Inizializza la torque
torque = zeros([3,1]);
torque_contribution = [0;0;0];

if eclipse_flag ~= 0
    sat_face_area = zeros(1, 10);

    panel_area = 0.200 * 0.610; % m^2
    
    sat_face_area(1) = 0.100 * 0.200;               % +Z Top face
    sat_face_area(2) = 0.300 * 0.200;               % +Y face
    sat_face_area(3) = 0.300 * 0.100;               % +X face
    sat_face_area(4) = 0.100 * 0.200;               % -Z Bottom face
    sat_face_area(5) = 0.300 * 0.200;               % -Y face
    sat_face_area(6) = 0.300 * 0.200;               % -X
    sat_face_area(7) = panel_area;                  % +Z +X
    sat_face_area(8) = panel_area;                  % +Z -X
    sat_face_area(9) = panel_area;                  % -Z +X
    sat_face_area(10) = panel_area;                 % -Z -X
    
    CP_positions = zeros(3, 10);
    CP_positions(:,1) = [0, 0, 0.190];   % +Z
    CP_positions(:,2) = [0, 0.050, 0.040];   % +Y
    CP_positions(:,3) = [0.100, 0, 0.040];   % +X
    CP_positions(:,4) = [0, 0, -0.110];  % -Z
    CP_positions(:,5) = [0, -0.050, 0.040];     % -Y
    CP_positions(:,6) = [-0.100, 0, 0.040];     % -X
    CP_positions(:,7) = [0, 0.355, 0.110];      % +Z +X
    CP_positions(:,8) = [0, 0.355, 0.110];      % -Z +X
    CP_positions(:,9) = [0, -0.355, 0.110];     % +Z -X
    CP_positions(:,10) = [0, -0.355, 0.110];   % -Z -X
    
    C_d_coeff = zeros(1, 10);
    C_d_coeff(1) = 1.5;             % +Z
    C_d_coeff(2) = 1.5;             % +Y
    C_d_coeff(3) = 1.5;             % +X
    C_d_coeff(4) = 1.5;             % -Z
    C_d_coeff(5) = 1.5;             % -Y
    C_d_coeff(6) = 1.5;             % -X
    C_d_coeff(7) = 1;           % pannello dx
    C_d_coeff(8) = 1;           % pannello sx
    C_d_coeff(9) = 1.5;
    C_d_coeff(10) = 1.5;
    
    
    faces = zeros(3, 10); %matrix of the faces normals
    faces(:,1) = [0, 0, 1];   % +Z
    faces(:,2) = [0, 1, 0];   % +Y
    faces(:,3) = [1, 0, 0];   % +X
    faces(:,4) = [0, 0, -1];  % -Z
    faces(:,5) = [0, -1, 0];  % -Y
    faces(:,6) = [-1, 0, 0];  % -X
    faces(:,7) = [0, 0, -1];   % -Z
    faces(:,8) = [0, 0, -1];   % -Z
    faces(:,9) = [0, 0, 1];   % +Z
    faces(:,10) = [0, 0, 1];   % +Z
    
    
    % Calcola direzione sole nel BRF
    Sdir_BRF_vec = R_ECIBRF * Sdir_ECI_vec;
    
    % Calcola torque per ogni faccia
    for i = 1:length(faces(1,:))
        
        % Controlla visibilità
        cos_theta = dot(Sdir_BRF_vec, faces(:,i));
    
        if cos_theta > cosd(180/2)
            area = sat_face_area(i);
            F_magnitude = P_sun * area * C_d_coeff(i) * cos_theta;
            
            F_vector = -1*F_magnitude * faces(:,i);
    
            % Calcola torque
            r_cp = CP_positions(:,i);
            torque_contribution = cross(r_cp, F_vector);
            torque = torque + torque_contribution;
        end
    end
    
end

== matlab function ExerciseModel_18072025/MEKF Performances/R(IRF->BRF) ==
  data: q input; R output
function R = R_by_q(q)

%% Description 
% This block provides the rotation matrix corresponding to the quaternion
% in input. THE SCALAR LAST CONVENTION IS USED FOR THE QUATERNION

%% INPUT 
% q -> 4x1 array (quaternion)
%% OUTPUT 
% R -> 3x3 matrix (rotation matrix)
q0 = q(4); 
q1 = q(1);
q2 = q(2);
q3 = q(3);

R = [q0^2+q1^2-q2^2-q3^2 2*q1*q2+2*q0*q3 2*q1*q3-2*q0*q2;
    2*q1*q2-2*q0*q3 q0^2-q1^2+q2^2-q3^2 2*q2*q3+2*q0*q1;
    2*q1*q3+2*q0*q2 2*q2*q3-2*q0*q1 q0^2-q1^2-q2^2+q3^2];
end

== matlab function ExerciseModel_18072025/External Disturbance Torques/AeroTorque in BRF/MATLAB Function ==
  data: z input; density output
% ATMOSPHERE calculates density for altitudes from sea level
% through 1000 km using exponential interpolation.
%wwwwwwwwwwwwwwwwwwwwwwwwwwwwwwwwwwwwwwwwwwwwwwwww
%function density = atmosphere(z)
%z[km]
function density = atmosphere(z)
%...Geometric altitudes (km):
h = ...
[ 0 25 30 40 50 60 70 ...
80 90 100 110 120 130 140 ...
150 180 200 250 300 350 400 ...
450 500 600 700 800 900 1000];
%...Corresponding densities (kg/m^3) from USSA76:
r = ...
[1.225 4.008e-2 1.841e-2 3.996e-3 1.027e-3 3.097e-4 8.283e-5 ...
1.846e-5 3.416e-6 5.606e-7 9.708e-8 2.222e-8 8.152e-9 3.831e-9 ...
2.076e-9 5.194e-10 2.541e-10 6.073e-11 1.916e-11 7.014e-12 2.803e-12 ...
1.184e-12 5.215e-13 1.137e-13 3.070e-14 1.136e-14 5.759e-15 3.561e-15];
%...Scale heights (km):
H = ...
[ 7.310 6.427 6.546 7.360 8.342 7.583 6.661 ...
5.927 5.533 5.703 6.782 9.973 13.243 16.322 ...
21.652 27.974 34.934 43.342 49.755 54.513 58.019 ...
60.980 65.654 76.377 100.587 147.203 208.020];
%...Handle altitudes outside of the range:

if z > 1000
z = 1000;
elseif z < 0
z = 0;
end

i=0;  %initialize i

%...Determine the interpolation interval:
for j = 1:27
if z >= h(j) && z < h(j+1)
i = j;
end
end
if z == 1000
i = 27;
end
%...Exponential interpolation:
density = r(i)*exp(-(z - h(i))/H(i));
end %atmosphere
% %wwwwwwwwwwwwwwwwwwwwwwwwwwwwwwwwwwwwwwwwwwwwwwwww
%

== matlab function ExerciseModel_18072025/Actuators/MATLAB Function ==
  data: Bdir_BRF_matrix_noise input; Bdir_meas_BRF output; B_BRF_matrix_noise input; Bvec_meas_BRF output
function [Bdir_meas_BRF, Bvec_meas_BRF] = fcn(Bdir_BRF_matrix_noise, B_BRF_matrix_noise)
% Should support variabile number of measurements
Bdir_meas_BRF = zeros(3,1);
Bvec_meas_BRF = zeros(3,1);
sum_directions = zeros(3,1);

dim = size(Bdir_BRF_matrix_noise); % number of rows and columns in the magnetic field measurements matrix
t = dim(2); % number of columns in the magnetic field measurements matrix

sum_directions = sum(Bdir_BRF_matrix_noise,2); % sum of the directions (taken from measurements)
sum_measurements = sum(B_BRF_matrix_noise,2); %sum of the measurements

for i = 1:3
     Bdir_meas_BRF(i) = sum_directions(i) / t; % arithmetic mean of the measured directions (taken from measurements)
     Bvec_meas_BRF(i) = sum_measurements(i) / t; % arithmetic mean of the measurements 

end

Bdir_meas_BRF = Bdir_meas_BRF / norm(Bdir_meas_BRF); % normalize

end

== matlab function ExerciseModel_18072025/External Disturbance Torques/Magnetic Torque/Earth magnetc Field/Earth magnetic field  ==
  data: r_ECEF input; B output; nmax input; mmax input; K input; G input; H input
function B = fcn(r_ECEF, nmax, mmax, K, G, H)

R_mean = 6371.2; % Mean radius for International Geomagnetic Reference Field
e1 = [1 0 0];
e2 = [0 1 0];
e3 = [0 0 1];

A = zeros(nmax+3, mmax+3);
ctilde = zeros(nmax+3,1);
stilde = zeros(nmax+3,1);

[A, ctilde, stilde] = recursion(r_ECEF, nmax, mmax);

rho = norm(r_ECEF);
r_vers = r_ECEF'/rho;

u = r_vers(3); % argumento of latitude
B = [0 0 0];

scalar = (R_mean/rho)^2;
ttilde = G;
b1 = ttilde;
b2 = ttilde;
b3 = ttilde;
br = ttilde;
for n=1:nmax
    
   scalar = scalar*R_mean/rho;
   
   i = n+1;
    for m =0:n 
        
        j = m+1;
        
        if m <= mmax
            ttilde(i,j) = G(i,j)*ctilde(j) + H(i,j)*stilde(j);
            
            b3(i,j) =  -ttilde(i,j)*A(i,j+1);
            
            br(i,j) = ttilde(i,j)*(u*A(i,j+1) + (n+m+1)*A(i,j));
            
            B = B + scalar*K(i,j)*(b3(i,j)*e3 + br(i,j)*r_vers);
        end 
        
    if ((m > 0) && (m <= mmax))
        
        b1(i,j) = -m*A(i,j)*(G(i,j)*ctilde(j-1) + H(i,j)*stilde(j-1));
        
        b2(i,j) = -m*A(i,j)*(H(i,j)*ctilde(j-1) - G(i,j)*stilde(j-1));
        
        B = B + scalar*K(i,j)*(b1(i,j)*e1 + b2(i,j)*e2);
    end 
    end 

end
end

function [A, ctilde, stilde] = recursion(r, nmax, mmax)
A = zeros(nmax+3, mmax+3);

R_m = norm(r);
rhat = r./R_m;
u = rhat(3);

A(1,1) = 1;
A(2,1) = u;
A(2,2) = 1;

ctilde = zeros(nmax+3,1);
stilde = zeros(nmax+3,1);

ctilde(1) = 1;
ctilde(2) = rhat(1);
stilde(1) = 0;
stilde(2) = rhat(2);

for n = 2:nmax
    i = n+1;
    
    A(i,i) = prod(1:2:(2*n-1));
    A(i,i-1) = u*A(i,i);
    
    if n<=nmax
        
        ctilde(i) = ctilde(2) * ctilde(i-1) - stilde(2) * stilde(i-1);
        stilde(i)  = stilde(2) * ctilde(i-1) + ctilde(2) * stilde(i-1);
        
    end
  for m = 0:n
      
    j=m+1;
    
    if (m < (n-1)) && (m <= (mmax+1))
        
      A(i,j)=((2*n - 1)*u*A((i-1),j) - (n+m-1)*A((i-2),j))/(n-m);
      
    end

  end
end 
end

== matlab function ExerciseModel_18072025/Performance Block /MATLAB Function ==
  data: DCM input; roll output; pitch output; yaw output
function [roll, pitch, yaw] = calc_angles(DCM)
%321 DCM ORF->BRF;
%Angles' computation from the rotation matrix 321;
pitch=asin(-DCM(1,3));          %pitch angle (beta);
roll=atan2(DCM(2,3),DCM(3,3));  %roll angle (alpha);
yaw=atan2(DCM(1,2),DCM(1,1));   %yaw angle (gamma);

end

== matlab function ExerciseModel_18072025/Sun direction in ECI ==
  data: t input; r_ECI input; Sdir_ECI output; ET0 input
function Sdir_ECI = fcn(t, r_ECI, ET0)

ET = ET0 + t;
coder.extrinsic('cspice_spkpos');
% Preallocazione necessaria perché Simulink non sa che output aspettarsi
R_ESun_ECI = zeros(3,1);

[R_ESun_ECI, ~] = cspice_spkpos('SUN', ET, 'J2000', 'NONE', 'EARTH'); % Sun position in ECI wrt earth

R_SatSun_ECI = R_ESun_ECI - r_ECI(:); % Sun position wrt the sat in ECI
Sdir_ECI = R_SatSun_ECI/norm(R_SatSun_ECI); % Sun direction wrt sat ECI
end

== matlab function ExerciseModel_18072025/Actuators/Magnetotorquers/MATLAB Function ==
  data: d_min input; d_max input; d input; d_eff output
function d_eff = fcn(d_min, d_max, d)

d_eff = zeros(size(d));

for i = 1:3     
        if abs(d(i)) > d_max
            d_eff(i) = sign(d(i))*d_max;
        else
            d_eff(i) = d(i);
        end
    end
end
